simulink model "num4"  (R2019a)
settings: Solver=VariableStepAuto  StartTime=0.0  StopTime=10.0  RelTol=1e-3
undefined symbols (not defined in the file): B, C
libraries: simulink x1
settings Model: Creator=julia  LastModifiedBy=julia

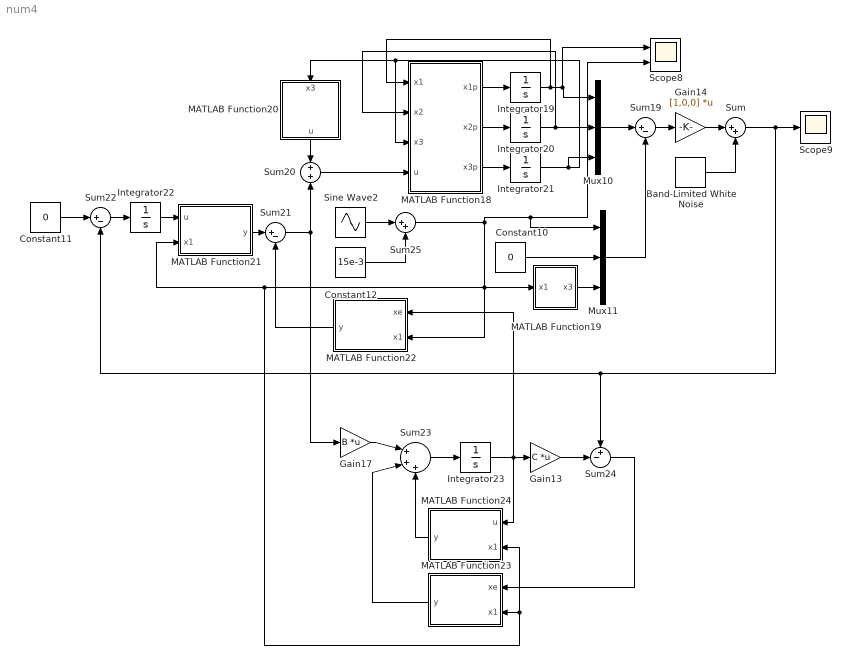
== system num4 ==
  Band-Limited White Noise : simulink/Sources/Band-Limited White Noise  Cov=[0.00000001]  Ts=0.1  seed=[23341]
  Constant10 : Constant  Value=0
  Constant11 : Constant  Value=0
  Constant12 : Constant  Value=15e-3
  Gain13 : Gain  Gain=C  Multiplication=Matrix(K*u)
  Gain14 : Gain  Gain=[1,0,0]  Multiplication=Matrix(K*u)
  Gain17 : Gain  Gain=B  Multiplication=Matrix(K*u)
  Integrator19 : Integrator  InitialCondition=5e-3
  Integrator{20..23} (4 alike) : Integrator
  MATLAB Function18 : MATLAB Function  TreatAsAtomicUnit=on
  MATLAB Function19 : MATLAB Function  TreatAsAtomicUnit=on
  MATLAB Function20 : MATLAB Function  TreatAsAtomicUnit=on
  MATLAB Function21 : MATLAB Function  TreatAsAtomicUnit=on
  MATLAB Function22 : MATLAB Function  TreatAsAtomicUnit=on
  MATLAB Function23 : MATLAB Function  TreatAsAtomicUnit=on
  MATLAB Function24 : MATLAB Function  TreatAsAtomicUnit=on
  Mux10 : Mux  Inputs=3
  Mux11 : Mux  Inputs=3
  Scope8 : Scope  NumInputPorts=2
  Scope9 : Scope
  Sine Wave2 : Sin  Amplitude=10e-3  Frequency=2  Phase=3.1+pi/2  SampleTime=0
  Sum : Sum  Inputs=|++
  Sum19 : Sum  Inputs=|+-
  Sum20 : Sum  Inputs=+|+
  Sum21 : Sum  Inputs=|+-
  Sum22 : Sum  Inputs=|+-
  Sum23 : Sum  Inputs=|+++
  Sum24 : Sum  Inputs=+-|
  Sum25 : Sum  Inputs=|++
  wires:
  Constant12/1 -> Sum25/2
  Sine Wave2/1 -> Sum25/1
  MATLAB Function22/1(y) -> Sum21/2
  Integrator22/1 -> MATLAB Function21/1(u)
  Constant11/1 -> Sum22/1
  Sum19/1 -> Gain14/1
  Sum21/1 -> Sum20/2, Gain17/1
  Sum22/1 -> Integrator22/1
  MATLAB Function21/1(y) -> Sum21/1
  MATLAB Function20/1(u) -> Sum20/1
  Sum20/1 -> MATLAB Function18/4(u)
  Mux11/1 -> Sum19/2
  MATLAB Function19/1(x3) -> Mux11/3
  Sum25/1 -> MATLAB Function22/2(x1), MATLAB Function19/1(x1), MATLAB Function23/2(x1), MATLAB Function24/2(x1), MATLAB Function21/2(x1), Mux11/1, Scope8/2
  Constant10/1 -> Mux11/2
  Mux10/1 -> Sum19/1
  Integrator21/1 -> Mux10/3, MATLAB Function18/3(x3), MATLAB Function20/1(x3)
  Integrator20/1 -> Mux10/2, MATLAB Function18/2(x2)
  Integrator19/1 -> Mux10/1, Scope8/1, MATLAB Function18/1(x1)
  MATLAB Function18/3(x3p) -> Integrator21/1
  MATLAB Function18/2(x2p) -> Integrator20/1
  MATLAB Function18/1(x1p) -> Integrator19/1
  Gain17/1 -> Sum23/1
  MATLAB Function24/1(y) -> Sum23/3
  MATLAB Function23/1(y) -> Sum23/2
  Sum23/1 -> Integrator23/1
  Integrator23/1 -> Gain13/1, MATLAB Function22/1(xe), MATLAB Function24/1(u)
  Gain13/1 -> Sum24/2
  Sum24/1 -> MATLAB Function23/1(xe)
  Gain14/1 -> Sum/1
  Sum/1 -> Sum24/1, Sum22/2, Scope9/1
  Band-Limited White Noise/1 -> Sum/2

== matlab function num4/MATLAB Function18 ==
  data: x1 input size=1; x1p output size=1; x2 input size=1; x3 input size=1; x2p output size=1; x3p output size=1; u input size=1
function [x1p,x2p,x3p] = planta(x1,x2,x3,u)
c=0.1;
m=0.01;
L=100e-3;
r=10;
g=9.81;

x1p=x2;
x2p=g-(c/m)*((x3^2)/x1);
x3p=-(r/L)*x3+(1/L)*u;

== matlab function num4/MATLAB Function19 ==
  data: x1 input size=1; x3 output size=1
function x3  = fcn(x1)
c=1
m=0.1
L=0.01
r=1
g=9.81

x3=sqrt((m*g*x1)/c);

== matlab function num4/MATLAB Function20 ==
  data: x3 input size=1; u output size=1
function u  = u(x3)
c=1
m=0.1
L=0.01
r=1
g=9.81

u=r*x3;

== matlab function num4/MATLAB Function21 ==
  data: u input size=1; x1 input size=1; y output size=1
function y = ki(u,x1)

k=-((1.0449e3)*x1)/(sqrt(0.981*x1));
y = k*u;

== matlab function num4/MATLAB Function22 ==
  data: xe input size=3; x1 input size=1; y output size=1
function y  = Kservo(xe,x1)

k1=-((2.9104e-15)*((6.1932e16)*x1+(1.6179e15)))/(sqrt(0.981*x1));
k2=-((9.0949e-17)*((1.6551e17)*x1+(5.3931e14)))/(sqrt(0.981*x1));
k3=-0.4;
k=[k1,k2,k3];
y = k*xe;

== matlab function num4/MATLAB Function23 ==
  data: xe input size=[1,1]; x1 input size=[1,1]; y output size=[3,1]
function y  = Kobs(xe,x1)

k1=2700;
k2=(1.8626e-11*((8.8934e16)*x1+5.2667e11))/x1;
k3=-(2.437e7*x1)/(sqrt(0.981*x1));
k=[k1;k2;k3];
y = k*xe;

== matlab function num4/MATLAB Function24 ==
  data: u input size=[3,1]; x1 input size=[1,1]; y output size=[3,1]
function y  = Amat(u,x1)

A=[0,1,0;(9.8100/x1),0,(-(20*sqrt(0.981*x1))/x1);0,0,-100];
y = A*u;
